simulink model "untitled"  (R2021a)
settings: Solver=VariableStepAuto  StartTime=0.0  StopTime=10.0  RelTol=1e-3
settings Model: Creator=zouxu  LastModifiedBy=zouxu

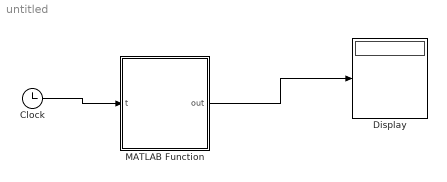
== system untitled ==
  Clock : Clock
  Display : Display
  MATLAB Function : MATLAB Function  TreatAsAtomicUnit=on
  wires:
  Clock/1 -> MATLAB Function/1(t)
  MATLAB Function/1(out) -> Display/1

== matlab function untitled/MATLAB Function ==
  data: out output; t input
function out = fcn(t)
x=0;
y=0;
z=0.5*t;
out=[x y z];
